simulink model "DISTURBANCE_MODEL_AUG20201"  (R2021b)
settings: Solver=FixedStepAuto  StartTime=0.0  StopTime=6000  FixedStep=1  RelTol=1e-3
values from neighbouring files (symbols this model uses):
  c_rk = 1.5    [test_parameters (1).m]
  Cd = 2.1    [test_parameters (1).m]
  coe = [a0;e0;Inc;RAAN_0;AoP;t0]    [test_parameters (1).m]
  day = 01    (= 1)    [test_parameters (1).m]
  E_prev = 0    [test_parameters (1).m]
  F_solar = 1366    [test_parameters (1).m]
  hours = 00    (= 0)    [test_parameters (1).m]
  I = [[37824169.23*10^-9 -25788.01*10^-9 32047.93*10^-9], ... (first row only)    [test_parameters (1).m]
  J2 = 1.083e-03    (= 0.001083)    [test_parameters (1).m]
  jd0 = JDnumber(year,month,day,hours,minutes,seconds)    [test_parameters (1).m]
  mass = 4    [test_parameters (1).m]
  minutes = 00    (= 0)    [test_parameters (1).m]
  month = 06    (= 6)    [test_parameters (1).m]
  mu_earth = 3.986e+14    (= 398600000000000)    [test_parameters (1).m]
  mu_moon = 4.913e+12    (= 4913000000000)    [test_parameters (1).m]
  mu_sun = 1.32712e+20    [test_parameters (1).m]
  q0 = [0 0 0 1]    [test_parameters (1).m]
  R_pm = [0.01 0.01 0.1]'    [test_parameters (1).m]
  RE = 6371800    [test_parameters (1).m]
  rho = 10^(-12)    (= 1e-12)    [test_parameters (1).m]
  S_norm = norm(S)    [test_parameters (1).m]
  seconds = 00    (= 0)    [test_parameters (1).m]
  speed_light_inverse = 1/299792458    (= 3.33564095198e-09)    [test_parameters (1).m]
  t0 = 0    [test_parameters (1).m]
  W0 = [0 0 0]    [test_parameters (1).m]
  w_earth = [0;0;7.2e-05]    [test_parameters (1).m]
  wc_drag_area = 0.042    [test_parameters (1).m]
  wc_solar_area = 0.12    [test_parameters (1).m]
  year = 2024    [test_parameters (1).m]
undefined symbols (not defined in the file or in its folder): IAU, magnitude, v0, WMM2020, x_dim, y_dim, z_dim
libraries: vrlib x12, aerolibtransform2 x2, dspmtrx3 x1, sharedtransform x1, aerolibgravity2 x1
settings Model: Creator=Owner  LastModifiedBy=mluser
settings SolverCC: AlgebraicLoopSolver=TrustRegion
settings DebuggingCC: SFMachineParentedDataDiag=warning
settings SFSimCC: CustomCodeUndefinedFunction=UseInterfaceOnly

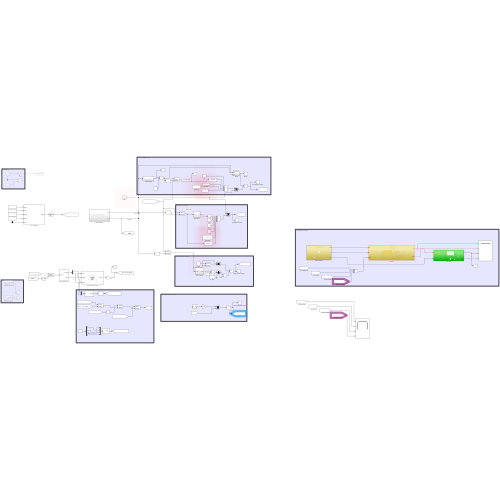
[thumbnail: Simulink's stored preview of the top-level diagram]
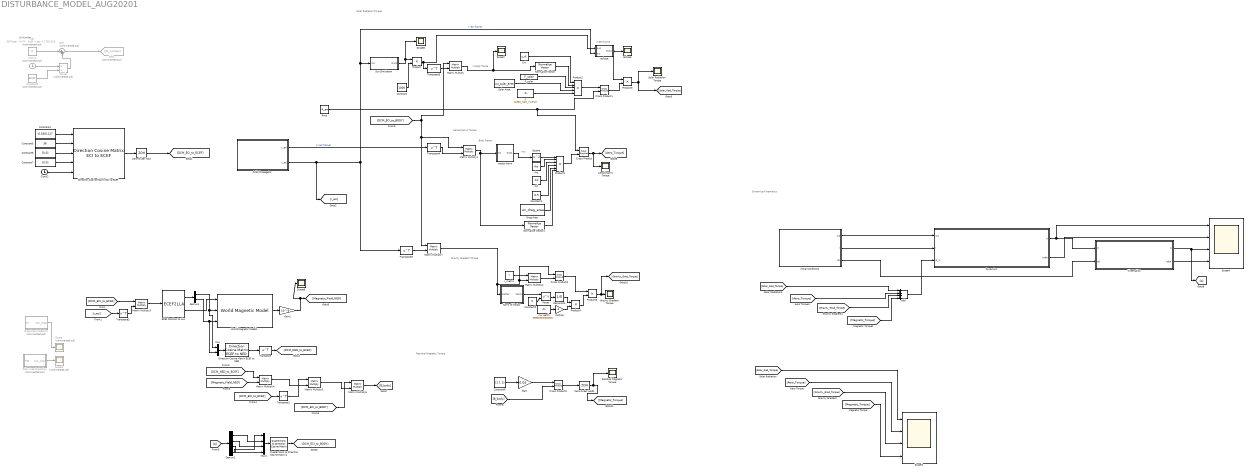
== system DISTURBANCE_MODEL_AUG20201 ==
  note: JD Number
  note: Dynamics/Kinematics
  note: Residual Magnetic Torque
  note: Gravity Gradient Torque
  note: Solar Radiation Torque
  note: Aerodynamic Torque
  note: Body frame
  note: in body frame
  note: Vsc
  note: in ECI frame
  Add : Sum  Inputs=++++
  Aerodynamic Torque : Scope
  "Cd " : Constant  Value=Cd
  Clock1 : Clock  Commented=on
  Clock2 : Clock
  Constant : Constant  Value=1000
  Constant1 : Constant  Value=0.5
  Constant2 : Constant  Value=5
  Constant3 : Constant  Commented=on  Value=8600  SampleTime=1
  Constant4 : Constant  Value=-0.0301117  SampleTime=1
  Constant5 : Constant  Value=36  SampleTime=1
  Constant6 : Constant  Value=[0,0]  SampleTime=1
  Constant7 : Constant  Value=[0,0]  SampleTime=1
  Constant8 : Constant  Value=[1 1 1]
  Crk : Constant  Value=c_rk
  Cross Product{,1..3} (4 alike) : vrlib/Utilities/Cross Product
  Demux1 : Demux  Outputs=2
  Demux2 : Demux
  Direction Cosine Matrix ECEF to NED : aerolibtransform2/Direction Cosine Matrix ECEF to NED
      settings: SourceProductBaseCode=AE
  Direction Cosine Matrix ECI to ECEF : aerolibtransform2/Direction Cosine Matrix ECI to ECEF  red=IAU-2000/2006  year=2024  month=June  day=1  hour=0  min=0  sec=0  deltaT=Sec  errorflag=Error  extraparamflag=on
      settings: AttributesFormatString=%<red>  SourceProductBaseCode=AE
  Divide : Product  Commented=on  Inputs=*/
  Drag Area : Constant  Value=wc_drag_area
  Drag Area Projection : Subsystem  Commented=on
  Dynamics : Subsystem
  ECEF Position to LLA : ECEF2LLA
  Eclipse : Scope
  F_solar : Constant  Value=F_solar
  Gain : Gain  Gain=0.04
  Gain1 : Gain  Gain=10^-9
  Goto : Goto  Commented=on  GotoTag=JD_number
  Gravity Gradient Torque : Scope
  I_matrix : Constant  Value=I
  Initial Conditions : Subsystem
  Kinematics : Subsystem
  Matrix Multiply{,1..7} (8 alike) : Product  Multiplication=Matrix(*)
  Multiply : Gain  Gain=3
  Mux : Mux  Inputs=2
  Mux1 : Mux
  Norm of Vector : Subsystem
  Normalize Vector : vrlib/Utilities/Normalize Vector  maxzero=0
  Normalize Vector1 : vrlib/Utilities/Normalize Vector  maxzero=0
  Orbit Propagator : Subsystem
  Power : Math  Operator=pow  SaturateOnIntegerOverflow=on
  Product{,3..5} (4 alike) : Product
  Product1 : Product  Inputs=6
  Product2 : Product  Inputs=5
  Quaternions to Direction Cosine Matrix1 : sharedtransform/Quaternions to  Direction Cosine Matrix  aMode=aMode
      settings: SourceProductBaseCode=AE,PW,DR,MT,UV,VE
  Reciprocal : Product  Inputs=/
  Residual Magnetic Torque : Scope
  "Rmp " : Constant  Value=-R_pm
  Scope : Scope  Commented=on
  Scope1 : Scope  Commented=on
  Scope3 : Scope  NumInputPorts=4
  Scope4 : Scope  NumInputPorts=4
  Scope6 : Scope
  Scope7 : Scope
  Scope8 : Scope
  Solar Area : Constant  Value=wc_solar_area
  "Solar Area Projection " : Subsystem  Commented=on
  Solar Radiation Torque : Scope
  Square : Math  Operator=square  SaturateOnIntegerOverflow=on
  Sum : Sum  Commented=on  Inputs=|++
  "Sun Simulation " : Subsystem
  Transpose{,3..5} (4 alike) : Math  Operator=transpose  SignedPower=on  RndMeth=Zero  SaturateOnIntegerOverflow=on
  Transpose1 : Math  Operator=transpose  SaturateOnIntegerOverflow=on
  Transpose2 : Math  Operator=transpose  SaturateOnIntegerOverflow=on
  "Vector Norm " : Subsystem
  World Magnetic Model1 : aerolibgravity2/World Magnetic Model  model=WMM2020 (2020-2025)  customFile='WMM2020.COF'  units=Metric (MKS)  time_in=off  month=June  day=1  year=2024  action=Error  h_out=off  dec_out=off  inc_out=off  ti_out=off
      settings: SourceProductBaseCode=AE
  Zero-Order Hold : ZeroOrderHold
  Zero-Order Hold1 : ZeroOrderHold  SampleTime=-1
  c : Constant  Value=speed_light_inverse
  eclipse : Subsystem
  jd0 : Constant  Commented=on  Value=367*year - fix(7*(year + fix((month + 9)/12))/4) + fix(275*month/9) + day + 1721013.5  SampleTime=1
  mu_earth : Constant  Value=398600000000000
  rho : Constant  Value=rho
  wires:
  rho/1 -> Product1/2
  "Cd "/1 -> Product1/3
  Constant1/1 -> Product1/4
  "Vector Norm "/1(Out1) -> Square/1
  Square/1 -> Product1/1
  Product1/1 -> Cross Product/2
  Cross Product/1 -> Aerodynamic Torque/1, [Aero_Torque]
  Crk/1 -> Product2/1
  F_solar/1 -> Product2/3
  c/1 -> Product2/5
  Product2/1 -> Cross Product1/1
  "Rmp "/1 -> Cross Product1/2, Cross Product/1
  Normalize Vector1/1 -> Product1/6
  Orbit Propagator/2(r_eci) -> [r_eci], Transpose3/1, eclipse/2(s/c), "Sun Simulation "/1(In1)  "r (eci frame)"
  Drag Area/1 -> Product1/5
  "Sun Simulation "/1(Out1) -> Scope8/1, Product/1
  Cross Product1/1 -> Product3/2
  Orbit Propagator/1(v_eci) -> Transpose4/1  "V (eci frame)"
  Solar Area/1 -> Product2/4
  Constant/1 -> Product/2
  Product/1 -> Transpose5/1, eclipse/1(sun)
  Normalize Vector/1 -> Product2/2
  "Solar Area Projection "/1(Asc_solar) -> Scope1/1
  Drag Area Projection/1(Asc_drag) -> Scope/1
  Product3/1 -> [Solar_Rad_Torque], Solar Radiation Torque/1
  Matrix Multiply1/1 -> "Vector Norm "/1(In1), Normalize Vector1/1
  Matrix Multiply/1 -> Scope7/1, Normalize Vector/1
  Product5/1 -> [Gravity_Grad_Torque], Gravity Gradient Torque/1
  Product4/1 -> Product5/2
  Cross Product2/1 -> Product5/1
  Reciprocal/1 -> Product4/1
  Matrix Multiply2/1 -> Cross Product2/2
  Norm of Vector/1(Norm) -> Power/1
  mu_earth/1 -> Multiply/1
  Constant2/1 -> Power/2
  Power/1 -> Reciprocal/1
  Multiply/1 -> Product4/2
  Initial Conditions/1(w0) -> Dynamics/1(w0)
  Kinematics/1(q) -> [q], Scope4/3
  Initial Conditions/3(q0) -> Kinematics/2(q0)
  Initial Conditions/2(I) -> Dynamics/2(I)
  Dynamics/1(w) -> Scope4/1, Kinematics/1(w)
  Kinematics/2(qdot) -> Scope4/4
  Dynamics/2(wdot) -> Scope4/2
  jd0/1 -> Sum/1
  Clock1/1 -> Divide/1
  Sum/1 -> Goto/1
  Constant3/1 -> Divide/2
  Divide/1 -> Sum/2
  Direction Cosine Matrix ECI to ECEF/1 -> Zero-Order Hold/1
  Constant4/1 -> Direction Cosine Matrix ECI to ECEF/1
  Constant5/1 -> Direction Cosine Matrix ECI to ECEF/2
  Constant6/1 -> Direction Cosine Matrix ECI to ECEF/3
  Constant7/1 -> Direction Cosine Matrix ECI to ECEF/4
  Clock2/1 -> Direction Cosine Matrix ECI to ECEF/5
  Zero-Order Hold/1 -> [DCM_ECI_to_ECEF]
  ECEF Position to LLA/1 -> Demux1/1
  Demux1/1 -> Mux/1, World Magnetic Model1/2
  Demux1/2 -> Mux/2, World Magnetic Model1/3
  ECEF Position to LLA/2 -> World Magnetic Model1/1
  [DCM_ECI_to_ECEF] -> Matrix Multiply3/1
  Matrix Multiply3/1 -> ECEF Position to LLA/1
  World Magnetic Model1/1 -> Gain1/1
  Direction Cosine Matrix ECEF to NED/1 -> Transpose/1
  Mux/1 -> Direction Cosine Matrix ECEF to NED/1
  Transpose/1 -> [DCM_NED_to_ECEF]
  [Magnetic_Field_NED] -> Matrix Multiply4/2
  [DCM_NED_to_ECEF] -> Matrix Multiply4/1
  [DCM_ECI_to_ECEF] -> Transpose1/1
  Matrix Multiply5/1 -> Matrix Multiply6/2
  Matrix Multiply4/1 -> Matrix Multiply5/2
  Transpose1/1 -> Matrix Multiply5/1
  [q] -> Demux2/1
  Demux2/1 -> Mux1/2
  Demux2/2 -> Mux1/3
  Demux2/3 -> Mux1/4
  Demux2/4 -> Mux1/1
  Mux1/1 -> Quaternions to Direction Cosine Matrix1/1
  Quaternions to Direction Cosine Matrix1/1 -> [DCM_ECI_to_BODY]
  [DCM_ECI_to_BODY] -> Matrix Multiply6/1
  Matrix Multiply6/1 -> [B_body]
  Constant8/1 -> Gain/1
  Gain/1 -> Cross Product3/1
  [B_body] -> Cross Product3/2
  Cross Product3/1 -> Zero-Order Hold1/1
  Zero-Order Hold1/1 -> [Magnetic_Torque], Residual Magnetic Torque/1
  [r_eci] -> Transpose2/1
  Transpose2/1 -> Matrix Multiply3/2
  Gain1/1 -> Scope6/1, [Magnetic_Field_NED]
  eclipse/1(Out1) -> Product3/1, Eclipse/1
  Matrix Multiply7/1 -> Norm of Vector/1(Vector), Matrix Multiply2/2, Cross Product2/1
  [DCM_ECI_to_BODY] -> Matrix Multiply/1, Matrix Multiply7/1, Matrix Multiply1/1
  Transpose3/1 -> Matrix Multiply7/2
  Transpose4/1 -> Matrix Multiply1/2
  Transpose5/1 -> Matrix Multiply/2
  I_matrix/1 -> Matrix Multiply2/1
  [Solar_Rad_Torque] -> Scope3/1
  [Magnetic_Torque] -> Scope3/4
  [Aero_Torque] -> Scope3/2
  [Gravity_Grad_Torque] -> Scope3/3
  Add/1 -> Dynamics/3(G_in)
  [Aero_Torque] -> Add/2
  [Magnetic_Torque] -> Add/4
  [Solar_Rad_Torque] -> Add/1
  [Gravity_Grad_Torque] -> Add/3

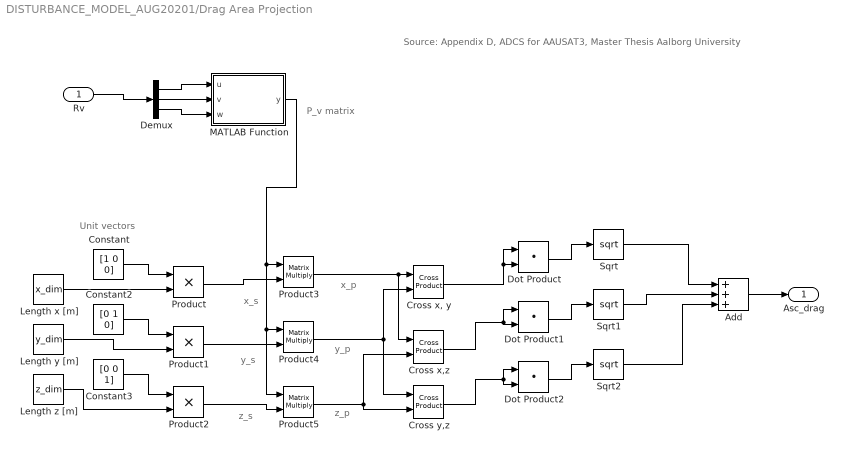
== system DISTURBANCE_MODEL_AUG20201/Drag Area Projection ==
  note: z_p
  note: y_p
  note: x_p
  note: P_v matrix
  note: z_s
  note: y_s
  note: x_s
  note: Source: Appendix D, ADCS for AAUSAT3, Master Thesis Aalborg University
  note: Unit vectors
  "Rv " : Inport
  Add : Sum  Inputs=+++
  Constant : Constant  Value=[1 0 0]
  Constant2 : Constant  Value=[0 1 0]
  Constant3 : Constant  Value=[0 0 1]
  "Cross x, y" : vrlib/Utilities/Cross Product
  Cross x,z : vrlib/Utilities/Cross Product
  Cross y,z : vrlib/Utilities/Cross Product
  Demux : Demux  Outputs=3
  Dot Product : DotProduct  InputSameDT=on  OutDataTypeStr=Inherit: Inherit via internal rule
  Dot Product1 : DotProduct  InputSameDT=on  OutDataTypeStr=Inherit: Inherit via internal rule
  Dot Product2 : DotProduct  InputSameDT=on  OutDataTypeStr=Inherit: Inherit via internal rule
  Length x [m] : Constant  Value=x_dim
  Length y [m] : Constant  Value=y_dim
  Length z [m] : Constant  Value=z_dim
  MATLAB Function : MATLAB Function  TreatAsAtomicUnit=on
  Product : Product
  Product1 : Product
  Product2 : Product
  Product3 : Product  Multiplication=Matrix(*)
  Product4 : Product  Multiplication=Matrix(*)
  Product5 : Product  Multiplication=Matrix(*)
  Sqrt : Sqrt  SaturateOnIntegerOverflow=on
  Sqrt1 : Sqrt  SaturateOnIntegerOverflow=on
  Sqrt2 : Sqrt  SaturateOnIntegerOverflow=on
  Asc_drag : Outport
  wires:
  Constant/1 -> Product/1
  Length x [m]/1 -> Product/2
  Constant2/1 -> Product1/1
  Length y [m]/1 -> Product1/2
  Constant3/1 -> Product2/1
  Length z [m]/1 -> Product2/2
  Product/1 -> Product3/2
  Product1/1 -> Product4/2
  Product2/1 -> Product5/2
  MATLAB Function/1(y) -> Product5/1, Product4/1, Product3/1
  Product3/1 -> Cross x,z/1, "Cross x, y"/1
  Product4/1 -> Cross y,z/1, "Cross x, y"/2
  Product5/1 -> Cross y,z/2, Cross x,z/2
  "Rv "/1 -> Demux/1
  Demux/1 -> MATLAB Function/1(u)
  Demux/2 -> MATLAB Function/2(v)
  Demux/3 -> MATLAB Function/3(w)
  Dot Product/1 -> Sqrt/1
  "Cross x, y"/1 -> Dot Product/1, Dot Product/2
  Cross x,z/1 -> Dot Product1/1, Dot Product1/2
  Dot Product1/1 -> Sqrt1/1
  Cross y,z/1 -> Dot Product2/1, Dot Product2/2
  Dot Product2/1 -> Sqrt2/1
  Sqrt2/1 -> Add/3
  Sqrt1/1 -> Add/2
  Sqrt/1 -> Add/1
  Add/1 -> Asc_drag/1

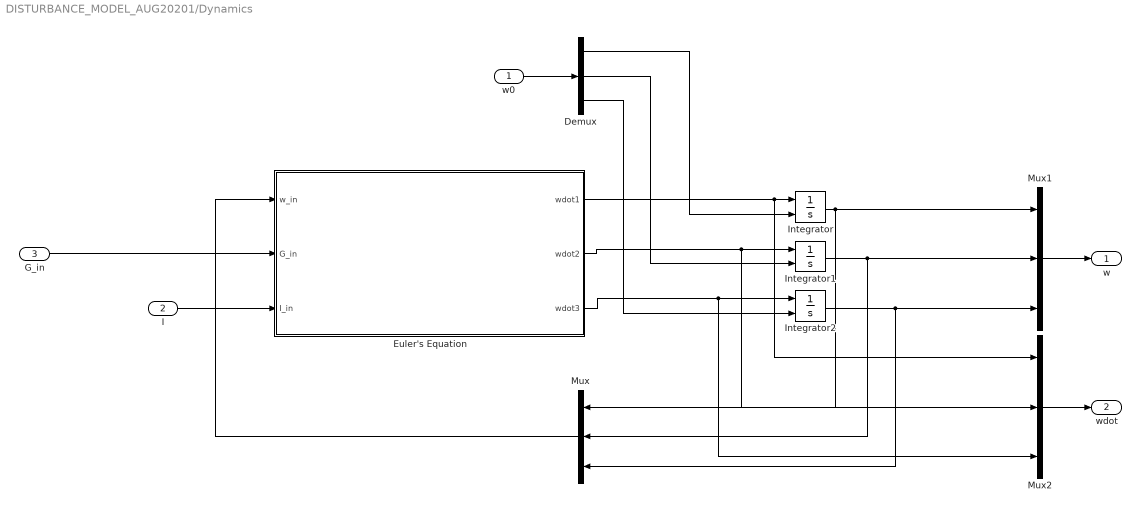
== system DISTURBANCE_MODEL_AUG20201/Dynamics ==
  w0 : Inport
  I : Inport  Port=2
  G_in : Inport  Port=3
  Demux : Demux  Outputs=3
  Euler's Equation : Subsystem
  Integrator : Integrator  InitialConditionSource=external
  Integrator1 : Integrator  InitialConditionSource=external
  Integrator2 : Integrator  InitialConditionSource=external
  Mux : Mux  Inputs=3
  Mux1 : Mux  Inputs=3
  Mux2 : Mux  Inputs=3
  w : Outport
  wdot : Outport  Port=2
  wires:
  Integrator/1 -> Mux/1, Mux1/1
  G_in/1 -> Euler's Equation/2(G_in)
  Euler's Equation/2(wdot2) -> Mux2/2, Integrator1/1
  Demux/1 -> Integrator/2
  Euler's Equation/1(wdot1) -> Mux2/1, Integrator/1
  Demux/3 -> Integrator2/2
  Integrator2/1 -> Mux/3, Mux1/3
  Euler's Equation/3(wdot3) -> Mux2/3, Integrator2/1
  Integrator1/1 -> Mux/2, Mux1/2
  Demux/2 -> Integrator1/2
  Mux/1 -> Euler's Equation/1(w_in)
  w0/1 -> Demux/1
  I/1 -> Euler's Equation/3(I_in)
  Mux1/1 -> w/1
  Mux2/1 -> wdot/1

== system DISTURBANCE_MODEL_AUG20201/Initial Conditions ==
  Extract Diagonal : dspmtrx3/Extract Diagonal
      settings: SourceProductBaseCode=DS
  I_in : Constant  Value=I
  q0_in : Constant  Value=q0
  w0_in : Constant  Value=W0
  w0 : Outport
  I : Outport  Port=2
  q0 : Outport  Port=3
  wires:
  w0_in/1 -> w0/1
  q0_in/1 -> q0/1
  I_in/1 -> Extract Diagonal/1
  Extract Diagonal/1 -> I/1

== system DISTURBANCE_MODEL_AUG20201/Kinematics ==
  w : Inport
  q0 : Inport  Port=2
  Integrator : Integrator  InitialConditionSource=external
  QDotSolver : MATLAB Function  TreatAsAtomicUnit=on
  q : Outport
  qdot : Outport  Port=2
  wires:
  w/1 -> QDotSolver/1(w)
  QDotSolver/1(qdot) -> qdot/1, Integrator/1
  q0/1 -> Integrator/2
  Integrator/1 -> q/1, QDotSolver/2(q)

== system DISTURBANCE_MODEL_AUG20201/Norm of Vector ==
  Vector : Inport
  Add : Sum  Inputs=+++
  Demux : Demux  Outputs=3
  Sqrt : Sqrt  SaturateOnIntegerOverflow=on
  square : Math  Operator=magnitude^2  SaturateOnIntegerOverflow=on
  square1 : Math  Operator=magnitude^2  SaturateOnIntegerOverflow=on
  square2 : Math  Operator=magnitude^2  SaturateOnIntegerOverflow=on
  Norm : Outport
  wires:
  square2/1 -> Add/3
  Vector/1 -> Demux/1
  Sqrt/1 -> Norm/1
  Add/1 -> Sqrt/1
  Demux/3 -> square2/1
  square1/1 -> Add/2
  Demux/2 -> square1/1
  Demux/1 -> square/1
  square/1 -> Add/1

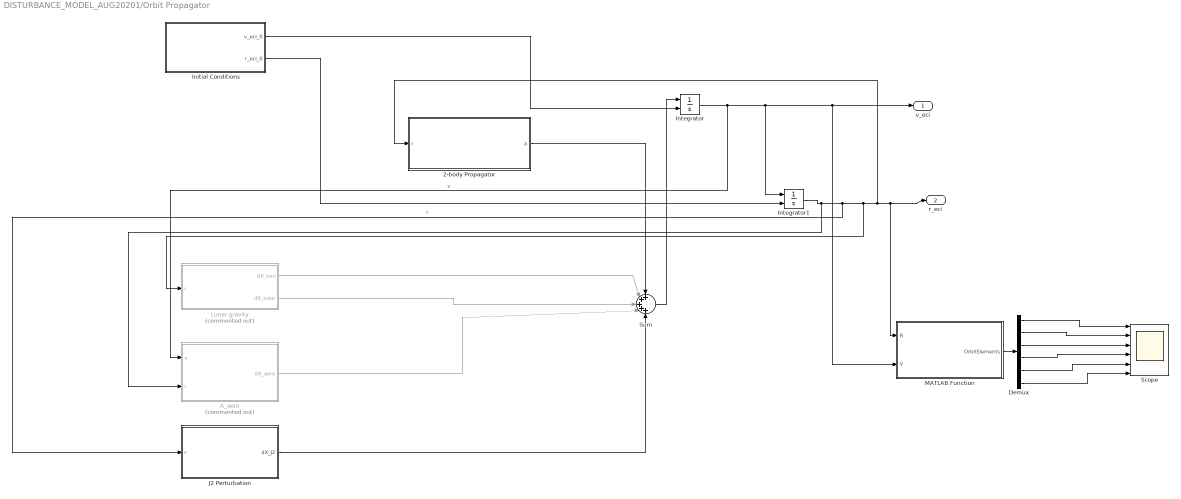
== system DISTURBANCE_MODEL_AUG20201/Orbit Propagator ==
  2-body Propagator : Subsystem
  A_aero : Subsystem  Commented=on
  Demux : Demux  Outputs=6
  Initial Conditions : Subsystem
  Integrator : Integrator  InitialConditionSource=external  InitialCondition=v0
  Integrator1 : Integrator  InitialConditionSource=external  InitialCondition=v0
  "J2 Perturbation " : Subsystem
  Lunar gravity : Subsystem  Commented=on
  MATLAB Function : MATLAB Function  TreatAsAtomicUnit=on
  Scope : Scope  NumInputPorts=6
  Sum : Sum  Inputs=+++++
  v_eci : Outport  VectorParamsAs1DForOutWhenUnconnected=off
  r_eci : Outport  Port=2  VectorParamsAs1DForOutWhenUnconnected=off
  wires:
  Integrator1/1 -> A_aero/2(r), "J2 Perturbation "/1(r), Lunar gravity/1(r), 2-body Propagator/1(r), MATLAB Function/1(R), r_eci/1  "r"
  Integrator/1 -> A_aero/1(v), Integrator1/1, MATLAB Function/2(V), v_eci/1  "v"
  Sum/1 -> Integrator/1
  Initial Conditions/1(v_eci_0) -> Integrator/2
  Initial Conditions/2(r_eci_0) -> Integrator1/2
  2-body Propagator/1(a) -> Sum/1
  "J2 Perturbation "/1(dX_J2) -> Sum/5
  A_aero/1(dX_aero) -> Sum/4
  MATLAB Function/1(OrbitElements) -> Demux/1
  Demux/1 -> Scope/1
  Demux/2 -> Scope/2
  Demux/3 -> Scope/3
  Demux/4 -> Scope/4
  Demux/5 -> Scope/5
  Demux/6 -> Scope/6
  Lunar gravity/2(dX_solar) -> Sum/3
  Lunar gravity/1(dX_luni) -> Sum/2

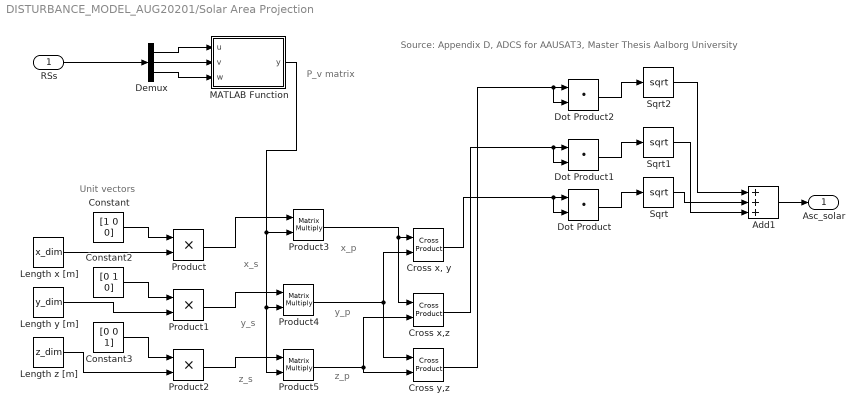
== system DISTURBANCE_MODEL_AUG20201/Solar Area Projection  ==
  note: z_p
  note: y_p
  note: x_p
  note: P_v matrix
  note: z_s
  note: y_s
  note: x_s
  note: Source: Appendix D, ADCS for AAUSAT3, Master Thesis Aalborg University
  note: Unit vectors
  "RSs " : Inport
  Add1 : Sum  Inputs=+++
  Constant : Constant  Value=[1 0 0]  VectorParams1D=off
  Constant2 : Constant  Value=[0 1 0]  VectorParams1D=off
  Constant3 : Constant  Value=[0 0 1]  VectorParams1D=off
  "Cross x, y" : vrlib/Utilities/Cross Product
  Cross x,z : vrlib/Utilities/Cross Product
  Cross y,z : vrlib/Utilities/Cross Product
  Demux : Demux  Outputs=3
  Dot Product : DotProduct  InputSameDT=on  OutDataTypeStr=Inherit: Inherit via internal rule
  Dot Product1 : DotProduct  InputSameDT=on  OutDataTypeStr=Inherit: Inherit via internal rule
  Dot Product2 : DotProduct  InputSameDT=on  OutDataTypeStr=Inherit: Inherit via internal rule
  Length x [m] : Constant  Value=x_dim
  Length y [m] : Constant  Value=y_dim
  Length z [m] : Constant  Value=z_dim
  MATLAB Function : MATLAB Function  TreatAsAtomicUnit=on
  Product : Product
  Product1 : Product
  Product2 : Product
  Product3 : Product  Multiplication=Matrix(*)
  Product4 : Product  Multiplication=Matrix(*)
  Product5 : Product  Multiplication=Matrix(*)
  Sqrt : Sqrt  SaturateOnIntegerOverflow=on
  Sqrt1 : Sqrt  SaturateOnIntegerOverflow=on
  Sqrt2 : Sqrt  SaturateOnIntegerOverflow=on
  Asc_solar : Outport
  wires:
  Constant/1 -> Product/1
  Length x [m]/1 -> Product/2
  Constant2/1 -> Product1/1
  Length y [m]/1 -> Product1/2
  Constant3/1 -> Product2/1
  Length z [m]/1 -> Product2/2
  Product/1 -> Product3/1
  Product1/1 -> Product4/1
  Product2/1 -> Product5/1
  MATLAB Function/1(y) -> Product5/2, Product4/2, Product3/2
  Product3/1 -> Cross x,z/1, "Cross x, y"/1
  Product4/1 -> Cross y,z/1, "Cross x, y"/2
  Product5/1 -> Cross y,z/2, Cross x,z/2
  "RSs "/1 -> Demux/1
  Demux/1 -> MATLAB Function/1(u)
  Demux/2 -> MATLAB Function/2(v)
  Demux/3 -> MATLAB Function/3(w)
  "Cross x, y"/1 -> Dot Product/2, Dot Product/1
  Dot Product/1 -> Sqrt/1
  Sqrt/1 -> Add1/2
  Dot Product1/1 -> Sqrt1/1
  Cross x,z/1 -> Dot Product1/2, Dot Product1/1
  Dot Product2/1 -> Sqrt2/1
  Cross y,z/1 -> Dot Product2/2, Dot Product2/1
  Sqrt1/1 -> Add1/3
  Sqrt2/1 -> Add1/1
  Add1/1 -> Asc_solar/1

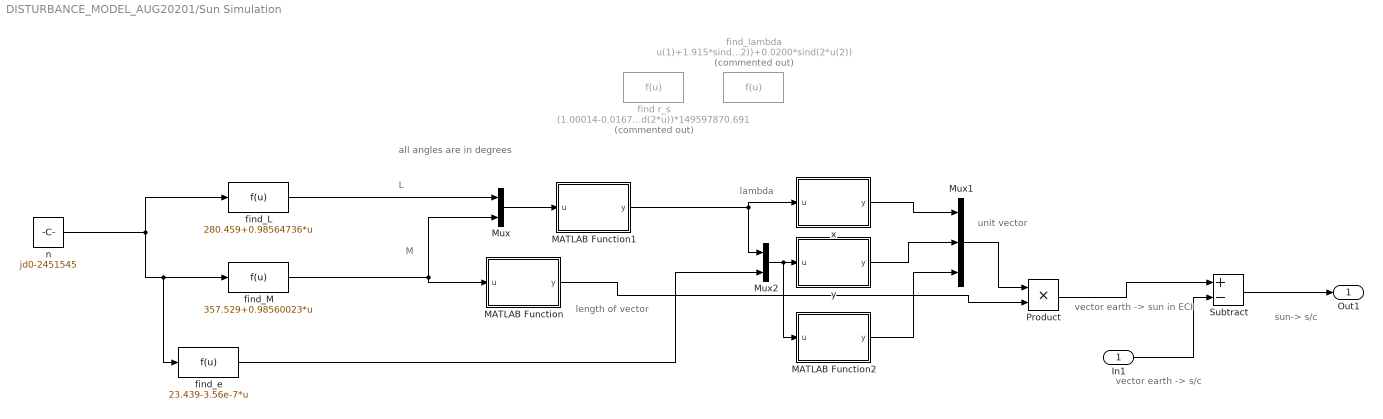
== system DISTURBANCE_MODEL_AUG20201/Sun Simulation  ==
  note: vector earth -> s/c
  note: sun-> s/c
  note: vector earth -> sun in ECI
  note: unit vector
  note: lambda
  note: all angles are in degrees
  note: length of vector
  note: L
  note: M
  In1 : Inport
  MATLAB Function : MATLAB Function  TreatAsAtomicUnit=on
  MATLAB Function1 : MATLAB Function  TreatAsAtomicUnit=on
  MATLAB Function2 : MATLAB Function  TreatAsAtomicUnit=on
  Mux : Mux  Inputs=2
  Mux1 : Mux  Inputs=3
  Mux2 : Mux  Inputs=2
  Product : Product
  Subtract : Sum  Inputs=+-
  find r_s : Fcn  Commented=on  Expr=(1.00014-0.01671*cosd(u)-0.000140*cosd(2*u))*149597870.691
  find_L : Fcn  Expr=280.459+0.98564736*u
  find_M : Fcn  Expr=357.529+0.98560023*u
  find_e : Fcn  Expr=23.439-3.56e-7*u
  find_lambda : Fcn  Commented=on  Expr=u(1)+1.915*sind(u(2))+0.0200*sind(2*u(2))
  n : Constant  Value=jd0-2451545
  "x " : MATLAB Function  TreatAsAtomicUnit=on
  "y " : MATLAB Function  TreatAsAtomicUnit=on
  Out1 : Outport
  wires:
  n/1 -> find_L/1, find_e/1, find_M/1
  find_L/1 -> Mux/1
  Mux/1 -> MATLAB Function1/1(u)
  MATLAB Function1/1(y) -> Mux2/1, "x "/1(u)
  "x "/1(y) -> Mux1/1
  find_e/1 -> Mux2/2
  Mux2/1 -> MATLAB Function2/1(u), "y "/1(u)
  "y "/1(y) -> Mux1/2
  MATLAB Function2/1(y) -> Mux1/3
  Mux1/1 -> Product/1
  MATLAB Function/1(y) -> Product/2
  Product/1 -> Subtract/1
  In1/1 -> Subtract/2
  Subtract/1 -> Out1/1
  find_M/1 -> Mux/2, MATLAB Function/1(u)

== system DISTURBANCE_MODEL_AUG20201/Vector Norm  ==
  In1 : Inport
  Add : Sum  Inputs=+++
  Demux : Demux  Outputs=3
  Square : Math  Operator=square  SaturateOnIntegerOverflow=on
  Square Root : Sqrt  SaturateOnIntegerOverflow=on
  Square1 : Math  Operator=square  SaturateOnIntegerOverflow=on
  Square2 : Math  Operator=square  SaturateOnIntegerOverflow=on
  Out1 : Outport
  wires:
  Demux/3 -> Square2/1
  Demux/1 -> Square/1
  Add/1 -> Square Root/1
  Square Root/1 -> Out1/1
  Square/1 -> Add/1
  Square2/1 -> Add/3
  Demux/2 -> Square1/1
  In1/1 -> Demux/1
  Square1/1 -> Add/2

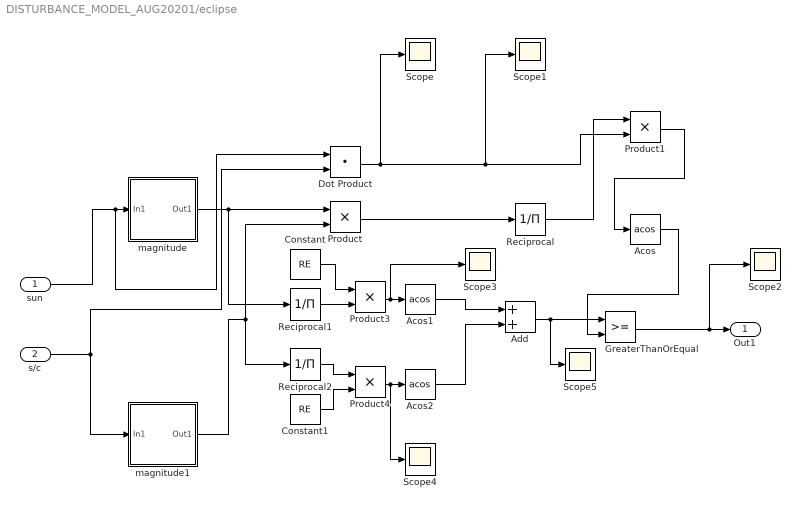
== system DISTURBANCE_MODEL_AUG20201/eclipse ==
  sun : Inport
  s/c : Inport  Port=2
  Acos : Trigonometry  Operator=acos
  Acos1 : Trigonometry  Operator=acos
  Acos2 : Trigonometry  Operator=acos
  Add : Sum
  Constant : Constant  Value=RE
  Constant1 : Constant  Value=RE
  Dot Product : DotProduct  InputSameDT=on  OutDataTypeStr=Inherit: Inherit via internal rule
  GreaterThanOrEqual : RelationalOperator  OutDataTypeStr=boolean  RndMeth=Simplest
  Product{,1,3..4} (4 alike) : Product
  Reciprocal : Product  Inputs=/
  Reciprocal1 : Product  Inputs=/
  Reciprocal2 : Product  Inputs=/
  Scope{,1..5} (6 alike) : Scope
  magnitude : Subsystem
  magnitude1 : Subsystem
  Out1 : Outport
  wires:
  sun/1 -> Dot Product/1, magnitude/1(In1)
  s/c/1 -> Dot Product/2, magnitude1/1(In1)
  magnitude/1(Out1) -> Reciprocal1/1, Product/1
  magnitude1/1(Out1) -> Reciprocal2/1, Product/2
  Add/1 -> Scope5/1, GreaterThanOrEqual/1
  GreaterThanOrEqual/1 -> Scope2/1, Out1/1
  Dot Product/1 -> Scope1/1, Product1/2, Scope/1
  Product/1 -> Reciprocal/1
  Reciprocal/1 -> Product1/1
  Constant/1 -> Product3/1
  Reciprocal1/1 -> Product3/2
  Reciprocal2/1 -> Product4/1
  Constant1/1 -> Product4/2
  Product3/1 -> Scope3/1, Acos1/1
  Product4/1 -> Scope4/1, Acos2/1
  Acos1/1 -> Add/1
  Acos2/1 -> Add/2
  Product1/1 -> Acos/1
  Acos/1 -> GreaterThanOrEqual/2

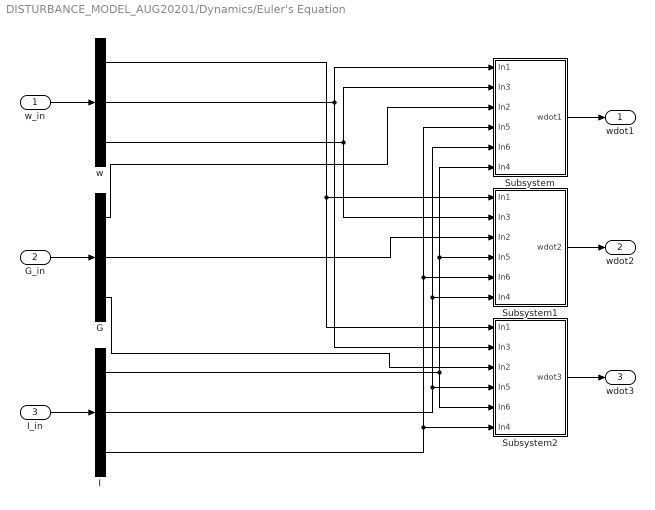
== system DISTURBANCE_MODEL_AUG20201/Dynamics/Euler's Equation ==
  w_in : Inport
  G_in : Inport  Port=2
  I_in : Inport  Port=3
  G : Demux  Outputs=3
  I : Demux  Outputs=3
  Subsystem : Subsystem
  Subsystem1 : Subsystem
  Subsystem2 : Subsystem
  w : Demux  Outputs=3
  wdot1 : Outport
  wdot2 : Outport  Port=2
  wdot3 : Outport  Port=3
  wires:
  Subsystem/1(wdot1) -> wdot1/1
  Subsystem1/1(wdot2) -> wdot2/1
  Subsystem2/1(wdot3) -> wdot3/1
  w_in/1 -> w/1
  G_in/1 -> G/1
  I_in/1 -> I/1
  w/2 -> Subsystem2/2(In3), Subsystem/1(In1)
  w/3 -> Subsystem1/2(In3), Subsystem/2(In3)
  w/1 -> Subsystem2/1(In1), Subsystem1/1(In1)
  G/1 -> Subsystem/3(In2)
  G/2 -> Subsystem1/3(In2)
  G/3 -> Subsystem2/3(In2)
  I/3 -> Subsystem2/6(In4), Subsystem1/5(In6), Subsystem/4(In5)
  I/2 -> Subsystem2/4(In5), Subsystem1/6(In4), Subsystem/5(In6)
  I/1 -> Subsystem2/5(In6), Subsystem1/4(In5), Subsystem/6(In4)

== system DISTURBANCE_MODEL_AUG20201/Orbit Propagator/2-body Propagator ==
  r : Inport
  Constant3 : Constant  Value=3
  Divide : Product  Inputs=*/
  Dot Product2 : DotProduct  InputSameDT=on  OutDataTypeStr=Inherit: Inherit via internal rule
  Gain : Gain  Gain=-mu_earth
  Power1 : Math  Operator=pow  SignedPower=on  SaturateOnIntegerOverflow=on
  Sqrt2 : Sqrt  SaturateOnIntegerOverflow=on
  a : Outport  VectorParamsAs1DForOutWhenUnconnected=off
  wires:
  Sqrt2/1 -> Power1/1
  r/1 -> Gain/1, Dot Product2/1, Dot Product2/2
  Power1/1 -> Divide/2  "r^3"
  Gain/1 -> Divide/1
  Constant3/1 -> Power1/2
  Dot Product2/1 -> Sqrt2/1
  Divide/1 -> a/1  "a"

== system DISTURBANCE_MODEL_AUG20201/Orbit Propagator/A_aero ==
  v : Inport
  r : Inport  Port=2
  A_aero : MATLAB Function  TreatAsAtomicUnit=on
  Constant : Constant  Value=Cd
  Constant1 : Constant  Value=mass
  Constant2 : Constant  Value=S_norm
  Constant3 : Constant  Value=w_earth
  Constant4 : Constant  Value=2.01e-12
  dX_aero : Outport  VectorParamsAs1DForOutWhenUnconnected=off
  wires:
  v/1 -> A_aero/2(v)
  Constant/1 -> A_aero/3(Cd)
  A_aero/1(dX_aero) -> dX_aero/1
  Constant1/1 -> A_aero/5(m)
  Constant2/1 -> A_aero/4(S)
  r/1 -> A_aero/1(r)
  Constant3/1 -> A_aero/7(w_earth)
  Constant4/1 -> A_aero/6(rho)

== system DISTURBANCE_MODEL_AUG20201/Orbit Propagator/Initial Conditions ==
  Constant : Constant  Value=coe
  Constant1 : Constant  Value=mu_earth
  Constant2 : Constant  Value=t0
  Constant3 : Constant  Value=E_prev
  MATLAB Function : MATLAB Function  TreatAsAtomicUnit=on
  v_eci_0 : Outport  VectorParamsAs1DForOutWhenUnconnected=off
  r_eci_0 : Outport  Port=2  VectorParamsAs1DForOutWhenUnconnected=off
  wires:
  Constant2/1 -> MATLAB Function/3(t)
  Constant1/1 -> MATLAB Function/2(mu)
  MATLAB Function/2(v_G) -> v_eci_0/1
  Constant3/1 -> MATLAB Function/4(E_prev)
  MATLAB Function/1(r_G) -> r_eci_0/1
  Constant/1 -> MATLAB Function/1(coe)

== system DISTURBANCE_MODEL_AUG20201/Orbit Propagator/J2 Perturbation  ==
  r : Inport
  Constant1 : Constant  Value=RE
  Constant2 : Constant  Value=J2
  Constant5 : Constant  Value=mu_earth
  J2 Perturbation : MATLAB Function  TreatAsAtomicUnit=on
  dX_J2 : Outport  VectorParamsAs1DForOutWhenUnconnected=off
  wires:
  Constant5/1 -> J2 Perturbation/4(mu)
  J2 Perturbation/1(dX_J2) -> dX_J2/1
  r/1 -> J2 Perturbation/1(r)
  Constant2/1 -> J2 Perturbation/3(J2)
  Constant1/1 -> J2 Perturbation/2(RE)

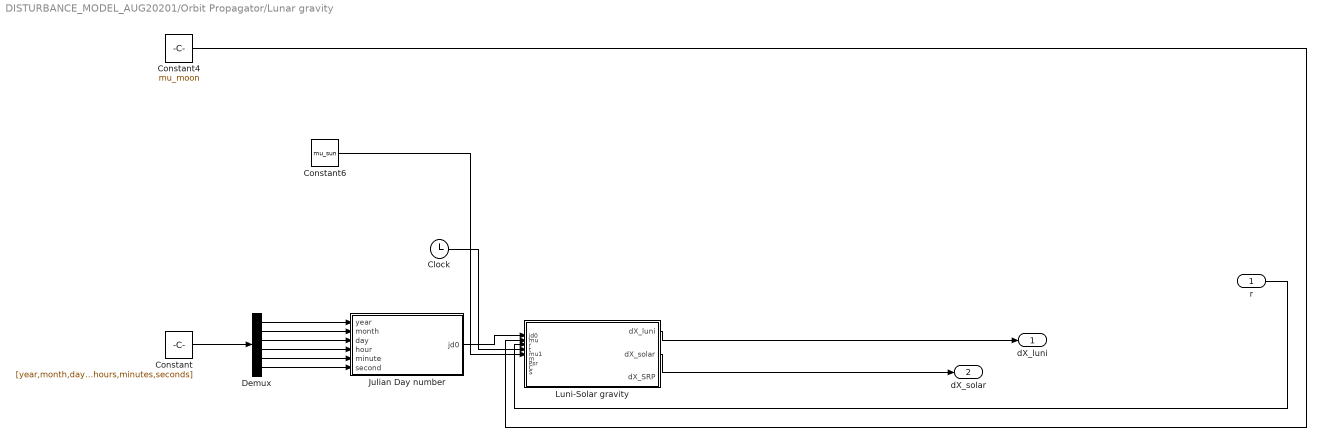
== system DISTURBANCE_MODEL_AUG20201/Orbit Propagator/Lunar gravity ==
  r : Inport
  Clock : Clock
  Constant : Constant  Value=[year,month,day,hours,minutes,seconds]
  Constant4 : Constant  Value=mu_moon
  Constant6 : Constant  Value=mu_sun
  Demux : Demux  Outputs=6
  Julian Day number : MATLAB Function  TreatAsAtomicUnit=on
  Luni-Solar gravity : MATLAB Function  TreatAsAtomicUnit=on
  dX_luni : Outport  VectorParamsAs1DForOutWhenUnconnected=off
  dX_solar : Outport  Port=2  VectorParamsAs1DForOutWhenUnconnected=off
  wires:
  Demux/6 -> Julian Day number/6(second)
  r/1 -> Luni-Solar gravity/3(r)
  Demux/4 -> Julian Day number/4(hour)
  Constant4/1 -> Luni-Solar gravity/2(mu)
  Demux/3 -> Julian Day number/3(day)
  Demux/1 -> Julian Day number/1(year)
  Demux/5 -> Julian Day number/5(minute)
  Julian Day number/1(jd0) -> Luni-Solar gravity/1(jd0)
  Demux/2 -> Julian Day number/2(month)
  Luni-Solar gravity/1(dX_luni) -> dX_luni/1
  Constant/1 -> Demux/1
  Clock/1 -> Luni-Solar gravity/4(t)
  Luni-Solar gravity/2(dX_solar) -> dX_solar/1
  Constant6/1 -> Luni-Solar gravity/5(mu1)

== system DISTURBANCE_MODEL_AUG20201/eclipse/magnitude ==
  In1 : Inport
  Dot Product : DotProduct  InputSameDT=on  OutDataTypeStr=Inherit: Inherit via internal rule
  Square Root : Sqrt  SaturateOnIntegerOverflow=on
  Out1 : Outport
  wires:
  Square Root/1 -> Out1/1
  Dot Product/1 -> Square Root/1
  In1/1 -> Dot Product/2, Dot Product/1

== system DISTURBANCE_MODEL_AUG20201/eclipse/magnitude1 ==
  In1 : Inport
  Dot Product : DotProduct  InputSameDT=on  OutDataTypeStr=Inherit: Inherit via internal rule
  Square Root : Sqrt  SaturateOnIntegerOverflow=on
  Out1 : Outport
  wires:
  Square Root/1 -> Out1/1
  Dot Product/1 -> Square Root/1
  In1/1 -> Dot Product/2, Dot Product/1

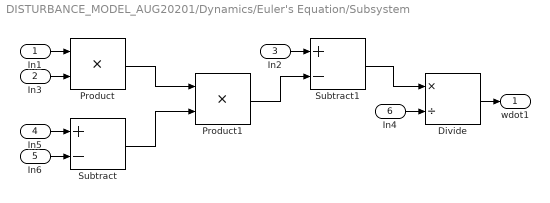
== system DISTURBANCE_MODEL_AUG20201/Dynamics/Euler's Equation/Subsystem ==
  In1 : Inport
  In3 : Inport  Port=2
  In2 : Inport  Port=3
  In5 : Inport  Port=4
  In6 : Inport  Port=5
  In4 : Inport  Port=6
  Divide : Product  Inputs=*/
  Product : Product
  Product1 : Product
  Subtract : Sum  Inputs=+-
  Subtract1 : Sum  Inputs=+-
  wdot1 : Outport
  wires:
  In3/1 -> Product/2
  In1/1 -> Product/1
  Product/1 -> Product1/1
  Subtract/1 -> Product1/2
  Product1/1 -> Subtract1/2
  Subtract1/1 -> Divide/1
  In5/1 -> Subtract/1
  In4/1 -> Divide/2
  Divide/1 -> wdot1/1
  In6/1 -> Subtract/2
  In2/1 -> Subtract1/1

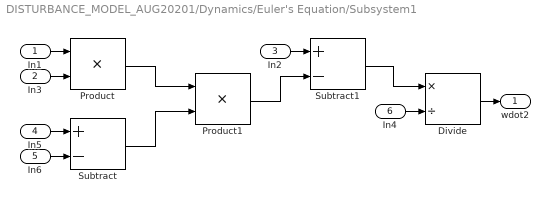
== system DISTURBANCE_MODEL_AUG20201/Dynamics/Euler's Equation/Subsystem1 ==
  In1 : Inport
  In3 : Inport  Port=2
  In2 : Inport  Port=3
  In5 : Inport  Port=4
  In6 : Inport  Port=5
  In4 : Inport  Port=6
  Divide : Product  Inputs=*/
  Product : Product
  Product1 : Product
  Subtract : Sum  Inputs=+-
  Subtract1 : Sum  Inputs=+-
  wdot2 : Outport
  wires:
  In3/1 -> Product/2
  In1/1 -> Product/1
  Product/1 -> Product1/1
  Subtract/1 -> Product1/2
  Product1/1 -> Subtract1/2
  Subtract1/1 -> Divide/1
  In5/1 -> Subtract/1
  In4/1 -> Divide/2
  Divide/1 -> wdot2/1
  In6/1 -> Subtract/2
  In2/1 -> Subtract1/1

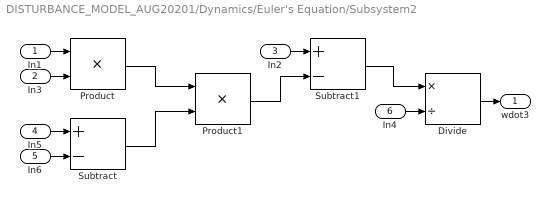
== system DISTURBANCE_MODEL_AUG20201/Dynamics/Euler's Equation/Subsystem2 ==
  In1 : Inport
  In3 : Inport  Port=2
  In2 : Inport  Port=3
  In5 : Inport  Port=4
  In6 : Inport  Port=5
  In4 : Inport  Port=6
  Divide : Product  Inputs=*/
  Product : Product
  Product1 : Product
  Subtract : Sum  Inputs=+-
  Subtract1 : Sum  Inputs=+-
  wdot3 : Outport
  wires:
  In3/1 -> Product/2
  In1/1 -> Product/1
  Product/1 -> Product1/1
  Subtract/1 -> Product1/2
  Product1/1 -> Subtract1/2
  Subtract1/1 -> Divide/1
  In5/1 -> Subtract/1
  In4/1 -> Divide/2
  Divide/1 -> wdot3/1
  In6/1 -> Subtract/2
  In2/1 -> Subtract1/1

== matlab function DISTURBANCE_MODEL_AUG20201/Orbit Propagator/MATLAB Function ==
  data: R input; OrbitElements output; V input
function OrbitElements = StateVectorToOrbitElements(R,V)
%{
INPUTS:
R: Radius Vector in ECI [km]
V: Velocity Vector in ECI [km/s]

OUTPUTS:
Struct called "OrbitElements" with the format:
    'a'     Semimajor Axis [m]
    'e'     Eccentricity Magnitude
    'i'     Inclination [deg]
    'w'     Argument of Periapse [deg]
    'RAAN'  Right Ascension of the Ascending Node [deg]
    'v'     True Anomaly [deg]
    'Alt'   Altitudes of Apogee and Perigee Respectively [km]
    'FPA'	Flight Path Angle [deg]
    'OE'    Orbit Energy [MJ/kg]
%}
%% Universal Variables
r_earth = 6378137; %m
u_earth = 3.986e+14; %m^3/s^2

%Inertial Axes
I = [1; 0; 0];
J = [0; 1; 0];
K = [0; 0; 1];

%% Determine Angular Momentum
H = cross(R,V); %m^2/s

%Orbit Energy
OE = norm(V)^2/2 - u_earth/norm(R); %m^2/s^2/kg => MJ/kg

%% Determination of Eccentricity
%Eccentricity Vector
e_vector = cross(V,H)/u_earth-R/norm(R);

%Scalor Eccentricity
e = norm(e_vector);

%% Semimajor Axis 
a = -u_earth/(norm(V)^2-(2*u_earth)/norm(R)); %km

%% Determine Inclination
i = acos(dot(K,H)/(norm(K)*norm(H))); %rad

%% Determine the Right Ascension of the Ascending Node
%Node Line Vector
N = cross(K,H);

%RAAN
if N(2) < 0
    RAAN = 2*pi - acos(dot(I,N)/(norm(I)*norm(N)));
else
    RAAN = acos(dot(I,N)/(norm(I)*norm(N)));
end

%% Determine The Argument of Periapse
if e_vector(3) < 0
    w = 2*pi - acos(dot(N,e_vector)/(norm(N)*norm(e_vector)));
else
    w = acos(dot(N,e_vector)/(norm(N)*norm(e_vector)));
end

%% Determine True Anomaly
if dot(R,V) < 0
    v = 2*pi - acos(dot(e_vector,R)/(norm(e_vector)*norm(R)));
else
    v = acos(dot(e_vector,R)/(norm(e_vector)*norm(R)));
end

%% Apogee & Perigee Altitudes
%Apogee
r_a = a*(1-e^2)/(1-e); %km
    h_a = r_a - r_earth; %km

%Perigee
r_p = a*(1-e^2)/(1+e); %km
    h_p = r_p - r_earth; %km

%% Flight Path Angle
phi_fpa = atan2(e*sin(v)/sqrt(1+2*e*cos(v)+e^2),...
               (1+e*cos(v))/sqrt(1+2*e*cos(v)+e^2));

%% Format Outputs
OrbitElements = [a;e;i*180/pi;w*180/pi;RAAN*180/pi;phi_fpa*180/pi];
%StateVectorToOrbitElements.m


end

== matlab function DISTURBANCE_MODEL_AUG20201/Sun Simulation /MATLAB Function2 ==
  data: u input; y output
function y = fcn(u)

y = sind(u(1))*sind(u(2));

== matlab function DISTURBANCE_MODEL_AUG20201/Drag Area Projection/MATLAB Function ==
  data: u input; y output; v input; w input
function y = fcn(u,v,w)
c=1/(norm(u))^2;

R_1=u;
R_2=v;
R_3=w;

matrix=zeros(3,3);

matrix(1,1)=R_2^2+R_3^2;
matrix(1,2)=-R_1*R_2;
matrix(1,3)=-R_1*R_3;

matrix(2,1)=-R_1*R_2;
matrix(2,2)=R_1^2+R_3^2;
matrix(2,3)=-R_2*R_3;

matrix(3,1)=-R_1*R_3;
matrix(3,2)=-R_2*R_3;
matrix(3,3)=R_1^2+R_2^2;

y=c*matrix;

end

== matlab function DISTURBANCE_MODEL_AUG20201/Sun Simulation /x  ==
  data: u input; y output
function y = fcn(u)

y = cosd(u);

== matlab function DISTURBANCE_MODEL_AUG20201/Sun Simulation /y  ==
  data: u input; y output
function y = fcn(u)

y = sind(u(1))*cosd(u(2));

== matlab function DISTURBANCE_MODEL_AUG20201/Kinematics/QDotSolver ==
  data: w input; qdot output; q input
function qdot  = QDotSolver(w,q)
    q1 = q(1);
    q2 = q(2);
    q3 = q(3);
    q4 = q(4);
    q_product = [
        q4, -q3, q2;
        q3, q4, -q1;
        -q2, q1, q4;
        -q1, -q2, -q3    
    ];
    qdot = 0.5*q_product*w;
end

== matlab function DISTURBANCE_MODEL_AUG20201/Orbit Propagator/J2 Perturbation /J2 Perturbation ==
  data: r input; dX_J2 output; RE input; J2 input; mu input
function dX_J2 = J2(r,RE,J2,mu)
rpp = norm(r);
xx = r(1); yy = r(2); zz = r(3);
fac = 3/2*J2*(mu/rpp^2)*(RE/rpp)^2;
dX_J2 = -fac*[(1 - 5*(zz/rpp)^2)*(xx/rpp) ...
(1 - 5*(zz/rpp)^2)*(yy/rpp) ...
(3 - 5*(zz/rpp)^2)*(zz/rpp)];
end

== matlab function DISTURBANCE_MODEL_AUG20201/Orbit Propagator/A_aero/A_aero ==
  data: r input; dX_aero output; v input; Cd input; S input; m input; rho input; w_earth input
function dX_aero = Aero(r,v,Cd,S,m,rho,w_earth)
sg = (Cd*S/2*m);
va = v - cross(w_earth,r);
v_a = norm(va);

dX_aero = sg*rho*(v_a^2)*(va/v_a);

end

== matlab function DISTURBANCE_MODEL_AUG20201/Orbit Propagator/Initial Conditions/MATLAB Function ==
  data: coe input; r_G output; mu input; t input; E_prev input; v_G output
function [r_G,v_G] = OrbMech(coe,mu, t, E_prev)
%ORBMECH models the orbital mechanics of the spacecraft
%   Assuming an ideal, non-perturbed orbit, the position of
%   the spacecraft (in the inertial frame) is determined, using the ISS
%   orbital elements

a = coe(1);e=coe(2);i=coe(3);raan=coe(4);w = coe(5);t0=coe(6);

% Solve for Eccentric Anomaly (E)
E_fun = @(E) E-e*sin(E) - sqrt(mu/a^3) * (t-t0);
E = fzero(E_fun,E_prev);

% Solve for True Anomaly (theta)
theta = 2*atan2(sqrt(1+e)*sin(E/2),sqrt(1-e)*cos(E/2));

% Compute SC position vector in the ECI frame (r_G)
r = a*(1 - e*cos(E));
ci=cos(i); co=cos(raan); cw=cos(w);si=sin(i); so=sin(raan); sw=sin(w);
C_PG = [cw*co-sw*ci*so, cw*so+sw*ci*co, sw*si;
        -sw*co-cw*ci*so, -sw*so+cw*ci*co, cw*si;
        si*so, -si*co, ci];
C_GP = C_PG';

% Compute SC position & velocity vector in the ECI frame
vel=sqrt(mu/a*(1-e^2))*[-sin(theta);e+cos(theta);0]; % Velocity vector of s/c in perifocal plane
r_G = C_GP * [r*cos(theta); r*sin(theta); 0];
v_G= C_GP* vel;

end

== matlab function DISTURBANCE_MODEL_AUG20201/Orbit Propagator/Lunar gravity/Julian Day number ==
  data: year input; jd0 output; month input; day input; hour input; minute input; second input
function jd0 = JDnumber(year,month,day,hour,minute,second)
% Calculates the JD number for a given year,month and day

j0 = 367*year - fix(7*(year + fix((month + 9)/12))/4) + fix(275*month/9) + day + 1721013.5; 

ut = hour + minute/60 + second/3600; % UTC time in hour format

jd0 = j0 + ut/24; % JD number calculation


end

== matlab function DISTURBANCE_MODEL_AUG20201/Orbit Propagator/Lunar gravity/Luni-Solar gravity ==
  data: jd0 input; dX_luni output; mu input; r input; t input; mu1 input; dX_solar output; m input; Psr input; C input; S input; dX_SRP output
function [dX_luni,dX_solar,dX_SRP] = LuniSolar(jd0,mu,r,t,mu1,m,Psr,C,S)
% Moon gravity contribution
jd_new = jd0 + t/86400;
R_moon = Lunargravity(jd_new);
R_ms = R_moon - r;
r_ms = norm(R_ms);
r_moon = norm(R_moon);

% Sun gravity contribution
[R_sun,u_sun] = Solargravity(jd_new);
lswitch = los(r,R_sun);
r_sun = norm(R_sun);
R_ss = R_sun - r;
r_ss = norm(R_ss);
q = dot(r,(2*R_sun - r))/r_sun^2;
Fq = q*(q^2 - 3*q +3)/(1 + sqrt(1-q));
%% SRP terms
psr = (lswitch*Psr*C*S)/m;

dX_luni = mu*((R_ms/r_ms^3) - (R_moon/r_moon^3));
dX_solar = (mu1/r_ss^3)*(Fq*R_sun - r);
dX_SRP = -psr*u_sun;
end

== matlab function DISTURBANCE_MODEL_AUG20201/Solar Area Projection /MATLAB Function ==
  data: u input; y output; v input; w input
function y = fcn(u,v,w)
c=1/(norm(u))^2;
R_1=u;
R_2=v;
R_3=w;

matrix=zeros(3,3);

matrix(1,1)=R_2^2+R_3^2;
matrix(1,2)=-R_1*R_2;
matrix(1,3)=-R_1*R_3;

matrix(2,1)=-R_1*R_2;
matrix(2,2)=R_1^2+R_3^2;
matrix(2,3)=-R_2*R_3;

matrix(3,1)=-R_1*R_3;
matrix(3,2)=-R_2*R_3;
matrix(3,3)=R_1^2+R_2^2;

y=c*matrix;

end

== matlab function DISTURBANCE_MODEL_AUG20201/Sun Simulation /MATLAB Function ==
  data: u input; y output
function y = fcn(u)



y = (1.00014-0.01671*cosd(u)-0.000140*cosd(2*u))*149597870.691;

== matlab function DISTURBANCE_MODEL_AUG20201/Sun Simulation /MATLAB Function1 ==
  data: u input; y output
function y = fcn(u)



y = u(1)+1.915*sind(u(2))+0.0200*sind(2*u(2));
